simulink model "sldemo_lct_sampletime"  (Simulink 7.6)
settings: Solver=FixedStepDiscrete  StartTime=0.0  StopTime=10.0  FixedStep=1  RelTol=1e-3
Description:
  | Fixed Point Parameters
settings Model: MinMaxOverflowLogging=MinMaxAndOverflow  Creator=The MathWorks Inc.  ExtModeAutoUpdateStatusClock=off  TunableVars=Kcs  TunableVarsStorageClass=ExportedGlobal
settings DataIOCC: SaveOutput=off  SaveTime=off  SignalLoggingName=logsOut
settings OptimizationCC: InlineParams=on  InlineInvariantSignals=on  InitFltsAndDblsToZero=on  EfficientFloat2IntCast=on
settings DebuggingCC: SaveWithParameterizedLinksMsg=none  SignalResolutionControl=TryResolveAllWithWarning  SolverPrmCheckMsg=none  MultiTaskDSMMsg=warning  MultiTaskCondExecSysMsg=none
settings RTWCC: GenerateReport=on  ProcessScript=grt_make_rtw_hook  LaunchReport=on  IncludeERTFirstTime=on
settings GRTTargetCC: TargetFcnLib=ansi_tfl_tmw.mat

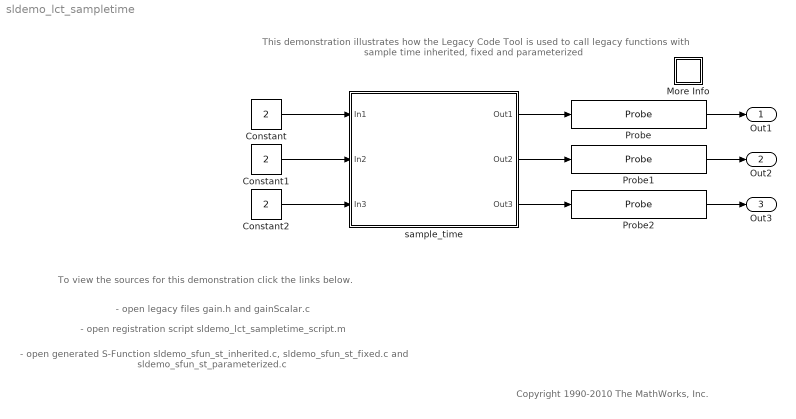
== system sldemo_lct_sampletime ==
  note: Copyright 1990-2010 The MathWorks, Inc.
  note: This demonstration illustrates how the Legacy Code Tool is used to
      | call legacy functions with sample time inherited, fixed and parameterized
  note: - open legacy files gain.h and gainScalar.c
  note: To view the sources for this demonstration
      | click the links below.
  note: - open registration script sldemo_lct_sampletime_script.m
  note: - open generated S-Function sldemo_sfun_st_inherited.c, sldemo_sfun_st_fixed.c
      |   and sldemo_sfun_st_parameterized.c
  Constant : Constant  Value=2  OutDataTypeStr=Inherit: Inherit via back propagation  SampleTime=1
  Constant1 : Constant  Value=2  OutDataTypeStr=Inherit: Inherit via back propagation  SampleTime=[2 1]
  Constant2 : Constant  Value=2  OutDataTypeStr=Inherit: Inherit via back propagation  SampleTime=[3 0]
  More Info : Subsystem
      settings: OpenFcn=showdemo('sldemo_lct_sampletime_script')
      mask Display: disp('?')
  Probe : Probe  ProbeWidth=off  ProbeComplexSignal=off
  Probe1 : Probe  ProbeWidth=off  ProbeComplexSignal=off
  Probe2 : Probe  ProbeWidth=off  ProbeComplexSignal=off
  sample_time : Subsystem
  Out1 : Outport
  Out2 : Outport  Port=2
  Out3 : Outport  Port=3
  wires:
  Constant/1 -> sample_time/1(In1)
  sample_time/1(Out1) -> Probe/1
  Constant1/1 -> sample_time/2(In2)
  Constant2/1 -> sample_time/3(In3)
  Probe/1 -> Out1/1
  Probe1/1 -> Out2/1
  Probe2/1 -> Out3/1
  sample_time/3(Out3) -> Probe2/1
  sample_time/2(Out2) -> Probe1/1

== system sldemo_lct_sampletime/More Info ==

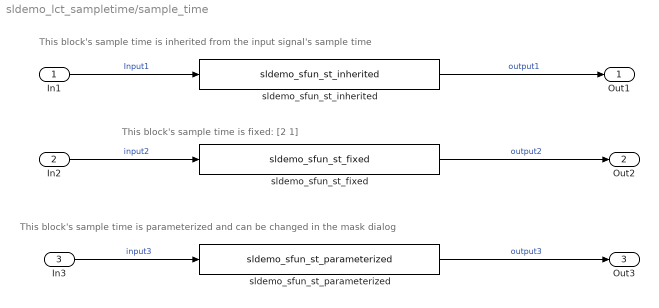
== system sldemo_lct_sampletime/sample_time ==
  note: This block's sample time is inherited from
      | the input signal's sample time
  note: This block's sample time is parameterized
      | and can be changed in the mask dialog
  note: This block's sample time is fixed: [2 1]
  In1 : Inport
  In2 : Inport  Port=2
  In3 : Inport  Port=3
  sldemo_sfun_st_fixed : S-Function  FunctionName=sldemo_sfun_st_fixed  Parameters=SParameter1  EnableBusSupport=off  mask(Legacy Function){SFunctionSpec=single y1 = gainScalar(single u1, single p1), SParameter1=2, ShowSpec=on}
      mask prompts: SParameter1 "P1:"; ShowSpec "Display function specification"
      mask help:
      | This block allows you to call the legacy functions specified by the following Legacy Code Tool definition:
      | def.SFunctionName = 'sldemo_sfun_st_fixed';
      | def.OutputFcnSpec = 'single y1 = gainScalar(single u1, single p1)';
      | def.HeaderFiles = {'gain.h'};
      | def.SourceFiles = {'gainScalar.c'};
      | def.IncPaths = {'sldemo_lct_src'};
      | def.SrcPaths = {'sldemo_lct_src'};
      | def.SampleTime = [2 1];
      mask Help: <p>This block was generated automatically by the Legacy Code Tool. For detailed help on this tool, call<a href="matlab:legacy_code('help')"> legacy_code('help')</a>.</p>
      mask CallbackString:
      | ||if strcmp(get_param(gcbh, 'ShowSpec'), 'on')
      |   set_param(gcbh, 'MaskDisplay', sprintf('fprintf(''%s'');', get_param(gcbh, 'SFunctionSpec')));
      | else
      |   set_param(gcbh, 'MaskDisplay', sprintf('fprintf(''%s'');', get_param(gcbh, 'FunctionName')));
      | end
      mask Display: fprintf('single y1 = gainScalar(single u1, single p1)');
  sldemo_sfun_st_inherited : S-Function  FunctionName=sldemo_sfun_st_inherited  Parameters=SParameter1  EnableBusSupport=off  mask(Legacy Function){SFunctionSpec=single y1 = gainScalar(single u1, single p1), SParameter1=2, ShowSpec=on}
      mask prompts: SParameter1 "P1:"; ShowSpec "Display function specification"
      mask help:
      | This block allows you to call the legacy functions specified by the following Legacy Code Tool definition:
      | def.SFunctionName = 'sldemo_sfun_st_inherited';
      | def.OutputFcnSpec = 'single y1 = gainScalar(single u1, single p1)';
      | def.HeaderFiles = {'gain.h'};
      | def.SourceFiles = {'gainScalar.c'};
      | def.IncPaths = {'sldemo_lct_src'};
      | def.SrcPaths = {'sldemo_lct_src'};
      mask Help: <p>This block was generated automatically by the Legacy Code Tool. For detailed help on this tool, call<a href="matlab:legacy_code('help')"> legacy_code('help')</a>.</p>
      mask CallbackString:
      | ||if strcmp(get_param(gcbh, 'ShowSpec'), 'on')
      |   set_param(gcbh, 'MaskDisplay', sprintf('fprintf(''%s'');', get_param(gcbh, 'SFunctionSpec')));
      | else
      |   set_param(gcbh, 'MaskDisplay', sprintf('fprintf(''%s'');', get_param(gcbh, 'FunctionName')));
      | end
      mask Display: fprintf('single y1 = gainScalar(single u1, single p1)');
  sldemo_sfun_st_parameterized : S-Function  FunctionName=sldemo_sfun_st_parameterized  Parameters=SParameter1, SampleTime  EnableBusSupport=off  mask(Legacy Function){SFunctionSpec=single y1 = gainScalar(single u1, single p1), SParameter1=2, SampleTime=3, ShowSpec=on}
      mask prompts: SParameter1 "P1:"; SampleTime "Sample time (-1 for inherited):"; ShowSpec "Display function specification"
      mask help:
      | This block allows you to call the legacy functions specified by the following Legacy Code Tool definition:
      | def.SFunctionName = 'sldemo_sfun_st_parameterized';
      | def.OutputFcnSpec = 'single y1 = gainScalar(single u1, single p1)';
      | def.HeaderFiles = {'gain.h'};
      | def.SourceFiles = {'gainScalar.c'};
      | def.IncPaths = {'sldemo_lct_src'};
      | def.SrcPaths = {'sldemo_lct_src'};
      | def.SampleTime = 'parameterized';
      mask Help: <p>This block was generated automatically by the Legacy Code Tool. For detailed help on this tool, call<a href="matlab:legacy_code('help')"> legacy_code('help')</a>.</p>
      mask CallbackString:
      | |||if strcmp(get_param(gcbh, 'ShowSpec'), 'on')
      |   set_param(gcbh, 'MaskDisplay', sprintf('fprintf(''%s'');', get_param(gcbh, 'SFunctionSpec')));
      | else
      |   set_param(gcbh, 'MaskDisplay', sprintf('fprintf(''%s'');', get_param(gcbh, 'FunctionName')));
      | end
      mask Display: fprintf('single y1 = gainScalar(single u1, single p1)');
  Out1 : Outport
  Out2 : Outport  Port=2
  Out3 : Outport  Port=3
  wires:
  In1/1 -> sldemo_sfun_st_inherited/1  "Input1"
  In2/1 -> sldemo_sfun_st_fixed/1  "input2"
  In3/1 -> sldemo_sfun_st_parameterized/1  "input3"
  sldemo_sfun_st_inherited/1 -> Out1/1  "output1"
  sldemo_sfun_st_fixed/1 -> Out2/1  "output2"
  sldemo_sfun_st_parameterized/1 -> Out3/1  "output3"
